simulink subsystem "th11_Tire"  (R2026a)
settings: Solver=VariableStepAuto
model mask{popup_leftRight=Left, tir_index=veh_index, Tire=Chassis.TireA1, VariantLabel=Chassis.TireA1.class.Value}
  mask prompts: popup_leftRight "Tire side"; tir_index "Tire index (tir file)"; Tire "Tire parameter struct"; VariantLabel "Variant label"
settings Model: Creator=th12-dv  LastModifiedBy=th12-dv

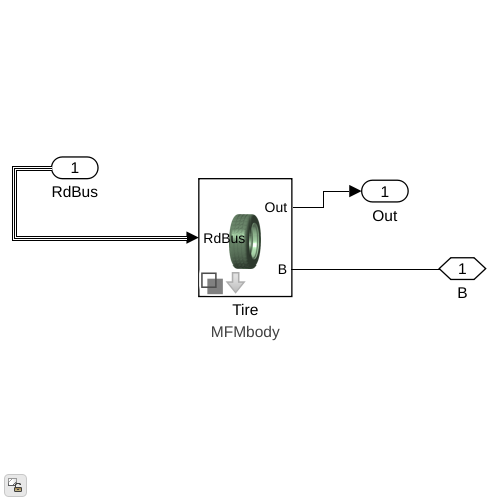
[thumbnail: Simulink's stored preview of the top-level diagram]
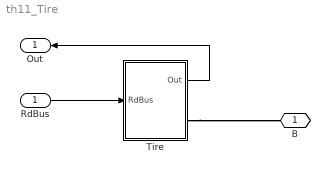
== system th11_Tire ==
  RdBus : Inport
  Tire : Subsystem  Tag=PublishSubsystem  Variant=on  VariantControlMode=label  VariantControl=Variant1  LabelModeActiveChoice=MFMbody  mask(Tire){popup_leftRight=Left, tir_index=tir_index, Tire=Tire, VariantLabel=VariantLabel}
      mask prompts: popup_leftRight "Left/Right"; tir_index "Tire Index"; Tire "Tire Parameters"; VariantLabel "Variant Label"
      mask help: Configurable tire model.
      mask init:
      | curblk = gcb;
      | 
      | % Set variant for this block 
      | set_param(curblk,'LabelModeActiveChoice',VariantLabel);
      | 
      | tir_variant = get_param(gcb,'ActiveVariant');
      | if (popup_leftRight == 1)
      |     rhs_tire = 1;
      |     if(strcmp(tir_variant,'MFEval'))
      |         set_param([gcb '/MFEval'],'tir_side','1 left');
      |         set_param([gcb '/MFEval'],'popup_leftRight','Left');
      |     elseif(strcmp(tir_variant,'Tire2x'))
      |         set_param([gcb '/Tire2x'],'popup_leftRight','Left');
      |     elseif(strcmp(tir_variant,'CFL'))
      |         set_param([gcb '/CFL'],'popup_leftRight','Left');
      |     elseif(strcmp(tir_variant,'Testrig_Post'))
      |         set_param([gcb '/Testrig Post'],'popup_leftRight','Left');
      |     elseif(strcmp(tir_variant,'Delft'))
      |         set_param([gcb '/Delft'],'tire_side_mode','(1xxx) left');
      |         set_param([gcb '/Delft'],'popup_leftRight','Left');
      |     elseif(strcmp(tir_variant,'MFSwift'))
      |         set_param([gcb '/MFSwift'],'tire_side_mode','(x1xxx) left');
      |         set_param([gcb '/MFSwift'],'popup_leftRight','Left');
      |     elseif(strcmp(tir_variant,'MFMbody'))
      |         set_param([gcb '/MFMbody'],'tire_side','Left');
      |         set_param([gcb '/MFMbody'],'popup_leftRight','Left');
      |     end
      | elseif (popup_leftRight == 2)
      |     rhs_tire = -1;
      |     if(strcmp(tir_variant,'MFEval'))
      |         set_param([gcb '/MFEval'],'tir_side','2 right');
      |         set_param([gcb '/MFEval'],'popup_leftRight','Right');
      |     elseif(strcmp(tir_variant,'Tire2x'))
      |         set_param([gcb '/Tire2x'],'popup_leftRight','Right');
      |     elseif(strcmp(tir_variant,'CFL'))
      |         set_param([gcb '/CFL'],'popup_leftRight','Right');
      |     elseif(strcmp(tir_variant,'Testrig_Post'))
      |         set_param([gcb '/Testrig Post'],'popup_leftRight','Right');
      |     elseif(strcmp(tir_variant,'Delft'))
      |         set_param([gcb '/Delft'],'tire_side_mode','(2xxx) right');
      |         set_param([gcb '/Delft'],'popup_leftRight','Right');
      |     elseif(strcmp(tir_variant,'MFSwift'))
      |         set_param([gcb '/MFSwift'],'tire_side_mode','(x2xxx) right');
      |         set_param([gcb '/MFSwift'],'popup_leftRight','Right');
      |     elseif(strcmp(tir_variant,'MFMbody'))
      |         set_param([gcb '/MFMbody'],'tire_side','Right');
      |         set_param([gcb '/MFMbody'],'popup_leftRight','Right');
      |         
      |     end
      | end
      settings: AttributesFormatString=%<ActiveVariant>
      mask TypeOptions popup_leftRight: Left | Right
      mask Display:
      | switch lower(get_param(gcb,'LabelModeActiveChoice'))
      |     case 'mfeval', image('sm_car_vehicle_tire_mfeval_IMAGE.png');
      |     case 'delft', image('sm_car_vehicle_tire_delft_IMAGE.png');
      |     case 'mfmbody', image('sm_car_vehicle_tire_mfmbody_IMAGE.png');
      |     case 'mfswift', image('sm_car_vehicle_tire_delft_IMAGE.png');
      |     case 'cpi', image('sm_car_vehicle_tire_delftcpi_IMAGE.png');
      |     case 'cfl', image('sm_car_vehicle_tire_cfl_IMAGE.png');
      |     case 'testrig_post', image('sm_car_vehicle_tire_testrig_IMAGE.png');
      |     case 'tire2x',
      |         switch lower(get_param([gcb '/Tire2x/Tire Inner'],'LabelModeActiveChoice'))
      |             case 'mfeval', image('sm_car_vehicle_tire_mfeval2x_IMAGE.png');
      |             case 'delft', image('sm_car_vehicle_tire_delft2x_IMAGE.png');
      |             case 'mfswift', image('sm_car_vehicle_tire_delft2x_IMAGE.png');
      |             case 'mfmbody', image('sm_car_vehicle_tire_mfmbody2x_IMAGE.png');
      |             case 'cfl', image('sm_car_vehicle_tire_cfl2x_IMAGE.png');
      |             case 'testrig', image('sm_car_vehicle_tire_testrig2x_IMAGE.png');
      |         end
      | end
  B : PMIOPort  Side=Left
  Out : Outport
  wires:
  Tire/1(" Out") -> Out/1
  RdBus/1 -> Tire/1(RdBus)
  connections:
  Tire/RConn1 -- B/RConn1

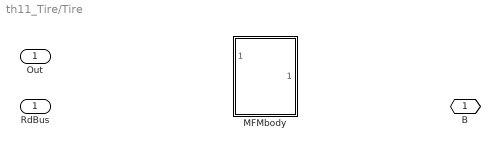
== system th11_Tire/Tire ==
  RdBus : Inport
  MFMbody : Subsystem  VariantControl=MFMbody  ReferencedSubsystem=th11_Tire_MF  tir_file=Tire.tirFile.Value  tire_side=Left  TireBody=Tire.TireBody  fcontactpatch=Tire.fContactPoint.Value  road_file=Tire.roadFile.Value  popup_leftRight=Left  clr_tyre=Visual.Tire.clr  opc_tyre=Visual.Tire.opc  clr_rim=Visual.Rim.clr  opc_rim=Visual.Rim.opc
  " B" : PMIOPort  Side=Right
  " Out" : Outport  VectorParamsAs1DForOutWhenUnconnected=off
